simulink model "calculate_trajectory"  (R2022a)
settings: Solver=VariableStepAuto  StartTime=0.0  StopTime=10.0  RelTol=1e-3
libraries: robotmaniplib x1, robotcorelib x1
settings Model: Creator=jaqueline.faino  LastModifiedBy=jaqueline.faino

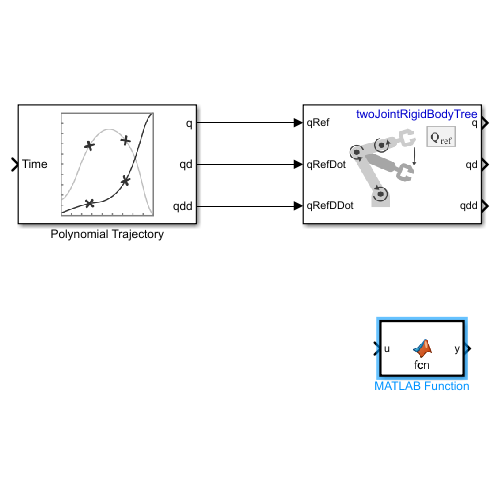
[thumbnail: Simulink's stored preview of the top-level diagram]
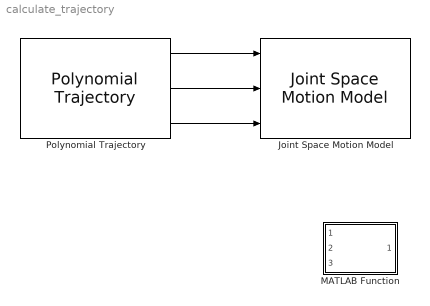
== system calculate_trajectory ==
  Joint Space Motion Model : robotmaniplib/Joint Space Motion Model  RigidBodyTree=twoJointRigidBodyTree  MotionType=Computed Torque Control  ProportionalGain=100  DerivativeGain=10  ErrorDynamicsSpecification=Damping Ratio / Natural Frequency  DampingRatio=1  NaturalFrequency=10  SettlingTime=0.59  Overshoot=0  ShowExternalForcePort=off  InitConfig=0  InitJointVel=0  SimulateUsing=Interpreted execution
      settings: SourceProductBaseCode=RO
  MATLAB Function : MATLAB Function  TreatAsAtomicUnit=on
  Polynomial Trajectory : robotcorelib/Polynomial Trajectory  WaypointSource=Internal  Waypoints=[ 0, 2, 1, 5, 0; -1, 3, 1, 4, 4 ]  TimePoints=[ 0, 1, 2, 3, 4 ]  TimeInterval=[ 1, 4 ]  Method=Cubic Polynomial  ParameterSource=Internal  VelocityBoundaryCondition=zeros( 2, 5 )  AccelerationBoundaryCondition=zeros( 2, 5 )  SimulateUsing=Interpreted execution
      settings: SourceProductBaseCode=RO,NV,RR,UV
  wires:
  Polynomial Trajectory/1 -> Joint Space Motion Model/1
  Polynomial Trajectory/2 -> Joint Space Motion Model/2
  Polynomial Trajectory/3 -> Joint Space Motion Model/3

== matlab function calculate_trajectory/MATLAB Function ==
  data: joint_angles_start input; trajectory output; joint_angles_goal input; num_steps input
function trajectory = calculate_trajectory(joint_angles_start, joint_angles_goal, num_steps)
    % Parâmetros: ângulos iniciais e finais, e o número de passos
    num_joints = length(joint_angles_start);
    trajectory = zeros(num_steps, num_joints);
    for i = 1:num_joints
        trajectory(:, i) = linspace(joint_angles_start(i), joint_angles_goal(i), num_steps);
    end
end
